simulink model "gm_sampleModel1695_sub"  (R2023a)
settings: Solver=VariableStepAuto  StartTime=0.0  StopTime=10.0  RelTol=1e-3
libraries: simulink x3
settings Model: Creator=user1  LastModifiedBy=user1
settings OptimizationCC: BlockReduction=off  ConditionallyExecuteInputs=off
settings DebuggingCC: InheritedTsInSrcMsg=none

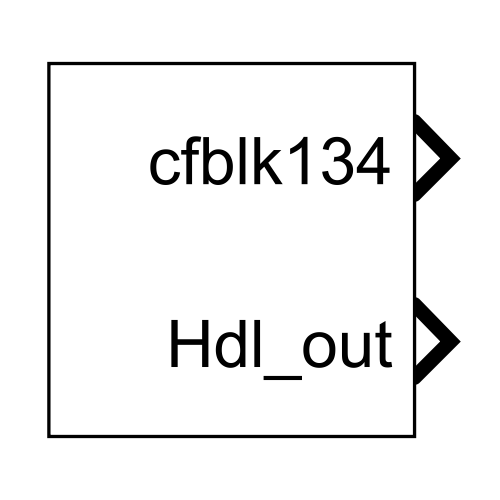
[thumbnail: Simulink's stored preview of the top-level diagram]
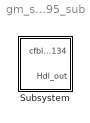
== system gm_sampleModel1695_sub ==
  Subsystem : Subsystem

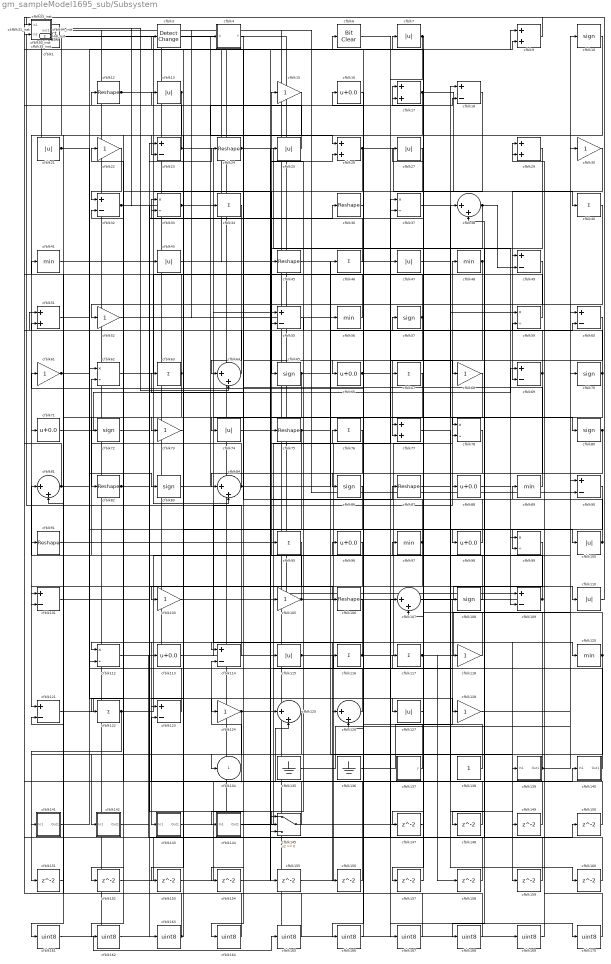
== system gm_sampleModel1695_sub/Subsystem ==
  cfblk1 : simulink/Logic and Bit Operations/Detect Increase  vinit=0.0  OutDataTypeStr=uint8
      settings: LibrarySourceBlock=|
      | hdlsllib/Logic and Bit
      | Operations/Detect
      | Increase
  cfblk{10,57,65,70,72,80,83,86,108} (9 alike) : Signum
  cfblk{7,13,21,25,27,43,47,74,100,110,115,127} (12 alike) : Abs  OutDataTypeStr=uint8  SaturateOnIntegerOverflow=off
  cfblk{18,23,32,49,55,60,69,90,101,109,114,121,123} (13 alike) : Sum  Inputs=+-  OutDataTypeStr=uint8
  cfblk102_inst : Subsystem
  cfblk{15,22,30,52,61,68,73,103,105,118,124,128} (12 alike) : Gain  OutDataTypeStr=uint8
  cfblk{12,24,36,45,75,82,87,91,106} (9 alike) : Reshape
  cfblk{38,64,81,84,107,125..126} (7 alike) : Sum  Inputs=|++  OutDataTypeStr=uint8
  cfblk{33,37,59,62,78,99,112} (7 alike) : Product  Inputs=*/  OutDataTypeStr=uint8  RndMeth=Zero  SaturateOnIntegerOverflow=on
  cfblk{16,66,71,88,96,98,113} (7 alike) : Bias  Bias=0.0  SaturateOnIntegerOverflow=off
  cfblk{34,40,46,63,67,76,95,116..117,122} (10 alike) : Sum  Inputs=+  OutDataTypeStr=uint8
  cfblk11_inst : Subsystem
  cfblk{41,48,56,89,97,120} (6 alike) : MinMax  OutDataTypeStr=uint8
  cfblk135 : Ground
  cfblk136 : Ground
  cfblk137 : Subsystem  mask(Counter Limited){uplimit=double(7), tsamp=double(-1)}
      mask prompts: uplimit "Simulink:masks:UpperLimit_MP"; tsamp "Simulink:masks:SampleTime_MP"
      mask help: Simulink:masks:CounterLimited_MD
      mask init:
      | nbits = double(8);
      | tsamp = double(-1);
      | uplimit = double(7);
  cfblk138 : Constant  OutDataTypeStr=uint8  SampleTime=-1
  cfblk139 : Subsystem
  cfblk140 : Subsystem
  cfblk141 : Subsystem
  cfblk142 : Subsystem
  cfblk143 : Subsystem
  cfblk144 : Subsystem
  cfblk145 : Switch  OutDataTypeStr=uint8  SaturateOnIntegerOverflow=off  InputSameDT=off
  cfblk{147..160} (14 alike) : Delay  SampleTime=1
  cfblk14_inst : Subsystem
  cfblk{161..170} (10 alike) : DataTypeConversion  OutDataTypeStr=uint8  SaturateOnIntegerOverflow=off  RndMeth=Floor
  cfblk{9,17,26,29,51,77} (6 alike) : Sum  OutDataTypeStr=uint8
  cfblk19_inst : Subsystem
  cfblk2 : Constant  Value=0  OutDataTypeStr=uint8  SampleTime=1
  cfblk28_inst : Subsystem
  cfblk3 : simulink/Logic and Bit Operations/Detect Change  vinit=0  OutDataTypeStr=uint8
      settings: LibrarySourceBlock=|
      | hdlsllib/Logic and Bit
      | Operations/Detect
      | Change
  cfblk31_inst : Subsystem
  cfblk35_inst : Subsystem
  cfblk4 : Subsystem  mask(Detect Fall Negative){vinit=double(0), InputProcessing=Elements as channels (sample based), OutDataTypeStr=uint8}
      mask prompts: vinit "Simulink:masks:InitialCondition_MP"; InputProcessing "Simulink:masks:InputProcessing_MP"; OutDataTypeStr "Simulink:masks:OutputDataType_MP"
      mask help: Simulink:masks:DetectFallNegative_MD
      mask init:
      | InputProcessing = 'Elements as channels (sample based)';
      | OutDataTypeStr = 'uint8';
      | vinit = double(0);
      mask TypeOptions InputProcessing: Simulink:masks:ColumnsAsChannelsFrameBased | Simulink:masks:ElementsAsChannelsSampleBased
      mask TypeOptions OutDataTypeStr: Simulink:masks:uint8 | Simulink:masks:boolean
      mask Display: fprintf('U < 0\n&  NOT\nU/z < 0')
  cfblk50_inst : Subsystem
  cfblk53_inst : Subsystem
  cfblk6 : simulink/Logic and Bit Operations/Bit Clear  iBit=0
      settings: LibrarySourceBlock=|
      | hdlsllib/Logic and Bit
      | Operations/Bit Clear
  cfblk94_inst : Subsystem
  cfblk134 : Outport  OutDataTypeStr=uint8  SampleTime=1  VectorParamsAs1DForOutWhenUnconnected=off
  Hdl_out : Outport  Port=2  OutDataTypeStr=uint8  SampleTime=1
  wires:
  cfblk1/1 -> cfblk84/2, cfblk121/1
  cfblk10/1 -> cfblk71/1
  cfblk100/1 -> cfblk48/1, cfblk89/1
  cfblk101/1 -> cfblk43/1
  cfblk102_inst/1(out1) -> cfblk47/1
  cfblk103/1 -> cfblk76/1
  cfblk105/1 -> cfblk81/1, cfblk15/1
  cfblk106/1 -> cfblk143/1(In1)
  cfblk107/1 -> cfblk110/1
  cfblk108/1 -> cfblk62/2
  cfblk109/1 -> cfblk91/1, Hdl_out/1
  cfblk11_inst/1(out1) -> cfblk109/1
  cfblk110/1 -> cfblk53_inst/1(in1)
  cfblk112/1 -> cfblk150/1
  cfblk113/1 -> cfblk88/1
  cfblk114/1 -> cfblk35_inst/2(in2)
  cfblk115/1 -> cfblk108/1, cfblk37/1
  cfblk116/1 -> cfblk78/2, cfblk112/1
  cfblk117/1 -> cfblk70/1, cfblk158/1
  cfblk118/1 -> cfblk33/1
  cfblk12/1 -> cfblk65/1, cfblk155/1
  cfblk120/1 -> cfblk31_inst/2(in2), cfblk142/1(In1)
  cfblk121/1 -> cfblk127/1
  cfblk122/1 -> cfblk151/1, cfblk97/1
  cfblk123/1 -> cfblk22/1
  cfblk124/1 -> cfblk134/1, cfblk117/1
  cfblk125/1 -> cfblk141/1(In1)
  cfblk126/1 -> cfblk3/1
  cfblk127/1 -> cfblk57/1
  cfblk128/1 -> cfblk30/1
  cfblk13/1 -> cfblk101/2, cfblk152/1
  cfblk135/1 -> cfblk10/1
  cfblk136/1 -> cfblk118/1
  cfblk137/1(y) -> cfblk96/1
  cfblk138/1 -> cfblk61/1
  cfblk139/1(Out1) -> cfblk90/1, cfblk75/1
  cfblk14_inst/1(out1) -> cfblk163/1
  cfblk140/1(Out1) -> cfblk62/1
  cfblk141/1(Out1) -> cfblk7/1
  cfblk142/1(Out1) -> cfblk140/1(In1)
  cfblk143/1(Out1) -> cfblk38/1
  cfblk144/1(Out1) -> cfblk46/1
  cfblk145/1 -> cfblk50_inst/2(in2)
  cfblk147/1 -> cfblk1/1
  cfblk148/1 -> cfblk51/2
  cfblk149/1 -> cfblk114/2
  cfblk15/1 -> cfblk23/2
  cfblk150/1 -> cfblk32/2
  cfblk151/1 -> cfblk121/2
  cfblk152/1 -> cfblk107/1
  cfblk153/1 -> cfblk125/2
  cfblk154/1 -> cfblk9/2
  cfblk155/1 -> cfblk60/1
  cfblk156/1 -> cfblk123/2
  cfblk157/1 -> cfblk17/1
  cfblk158/1 -> cfblk53_inst/2(in2)
  cfblk159/1 -> cfblk38/2
  cfblk16/1 -> cfblk66/1
  cfblk160/1 -> cfblk35_inst/1(in1)
  cfblk161/1 -> cfblk165/1
  cfblk162/1 -> cfblk95/1
  cfblk163/1 -> cfblk33/2, cfblk41/1
  cfblk164/1 -> cfblk14_inst/1(in1)
  cfblk165/1 -> cfblk14_inst/2(in2)
  cfblk166/1 -> cfblk6/1
  cfblk167/1 -> cfblk11_inst/2(in2)
  cfblk168/1 -> cfblk11_inst/1(in1)
  cfblk169/1 -> cfblk29/1
  cfblk17/1 -> cfblk69/2, cfblk103/1
  cfblk170/1 -> cfblk29/2
  cfblk18/1 -> cfblk45/1
  cfblk19_inst/1(out1) -> cfblk169/1
  cfblk2/1 -> cfblk64/2, cfblk4/1(U)
  cfblk21/1 -> cfblk9/1, cfblk124/1
  cfblk22/1 -> cfblk32/1
  cfblk23/1 -> cfblk12/1, cfblk156/1
  cfblk24/1 -> cfblk125/1, cfblk109/2
  cfblk25/1 -> cfblk28_inst/1(in1)
  cfblk26/1 -> cfblk73/1, cfblk40/1
  cfblk27/1 -> cfblk52/1
  cfblk28_inst/1(out1) -> cfblk56/1
  cfblk29/1 -> cfblk168/1
  cfblk3/1 -> cfblk26/1
  cfblk30/1 -> cfblk49/1
  cfblk31_inst/1(out1) -> cfblk90/2, cfblk28_inst/2(in2)
  cfblk32/1 -> cfblk126/1, cfblk106/1
  cfblk33/1 -> cfblk77/2, cfblk55/1, cfblk159/1, cfblk105/1
  cfblk34/1 -> cfblk64/1
  cfblk35_inst/1(out1) -> cfblk113/1
  cfblk36/1 -> cfblk16/1
  cfblk37/1 -> cfblk59/1
  cfblk38/1 -> cfblk55/2, cfblk49/2
  cfblk4/1(Y) -> cfblk164/1
  cfblk40/1 -> cfblk122/1
  cfblk41/1 -> cfblk98/1
  cfblk43/1 -> cfblk18/2
  cfblk45/1 -> cfblk78/1
  cfblk46/1 -> cfblk23/1
  cfblk47/1 -> cfblk80/1
  cfblk48/1 -> cfblk77/1, cfblk126/2
  cfblk49/1 -> cfblk114/1
  cfblk50_inst/1(out1) -> cfblk115/1
  cfblk51/1 -> cfblk83/1
  cfblk52/1 -> cfblk26/2
  cfblk53_inst/1(out1) -> cfblk34/1
  cfblk55/1 -> cfblk145/2
  cfblk56/1 -> cfblk102_inst/1(in1)
  cfblk57/1 -> cfblk19_inst/2(in2), cfblk67/1
  cfblk59/1 -> cfblk27/1
  cfblk6/1 -> cfblk167/1
  cfblk60/1 -> cfblk144/1(In1)
  cfblk61/1 -> cfblk100/1, cfblk128/1
  cfblk62/1 -> cfblk18/1
  cfblk63/1 -> cfblk94_inst/2(in2), cfblk82/1
  cfblk64/1 -> cfblk51/1
  cfblk65/1 -> cfblk101/1, cfblk139/1(In1)
  cfblk66/1 -> cfblk170/1, cfblk68/1
  cfblk67/1 -> cfblk123/1
  cfblk68/1 -> cfblk116/1
  cfblk69/1 -> cfblk94_inst/1(in1), cfblk147/1
  cfblk7/1 -> cfblk107/2, cfblk37/2
  cfblk70/1 -> cfblk81/2, cfblk74/1, cfblk25/1
  cfblk71/1 -> cfblk69/1
  cfblk72/1 -> cfblk36/1
  cfblk73/1 -> cfblk13/1
  cfblk74/1 -> cfblk120/1
  cfblk75/1 -> cfblk59/2, cfblk153/1
  cfblk76/1 -> cfblk86/1
  cfblk77/1 -> cfblk160/1
  cfblk78/1 -> cfblk166/1
  cfblk80/1 -> cfblk84/1, cfblk148/1
  cfblk81/1 -> cfblk50_inst/1(in1), cfblk99/2
  cfblk82/1 -> cfblk24/1, cfblk145/3
  cfblk83/1 -> cfblk17/2
  cfblk84/1 -> cfblk72/1, cfblk60/2
  cfblk86/1 -> cfblk145/1
  cfblk87/1 -> cfblk149/1
  cfblk88/1 -> cfblk99/1
  cfblk89/1 -> cfblk102_inst/2(in2)
  cfblk9/1 -> cfblk31_inst/1(in1)
  cfblk90/1 -> cfblk154/1
  cfblk91/1 -> cfblk87/1
  cfblk94_inst/1(out1) -> cfblk21/1
  cfblk95/1 -> cfblk161/1
  cfblk96/1 -> cfblk162/1
  cfblk97/1 -> cfblk19_inst/1(in1), cfblk112/2
  cfblk98/1 -> cfblk63/1
  cfblk99/1 -> cfblk157/1

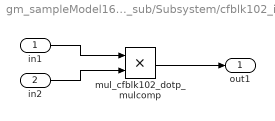
== system gm_sampleModel1695_sub/Subsystem/cfblk102_inst ==
  in1 : Inport  OutDataTypeStr=uint8  SampleTime=1
  in2 : Inport  Port=2  OutDataTypeStr=uint8  SampleTime=1
  mul_cfblk102_dotp_mulcomp : Product  Inputs=**  OutDataTypeStr=uint8  SampleTime=1
  out1 : Outport  OutDataTypeStr=uint8  SampleTime=1
  wires:
  in1/1 -> mul_cfblk102_dotp_mulcomp/1
  in2/1 -> mul_cfblk102_dotp_mulcomp/2
  mul_cfblk102_dotp_mulcomp/1 -> out1/1

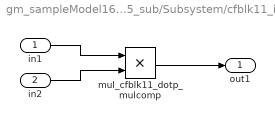
== system gm_sampleModel1695_sub/Subsystem/cfblk11_inst ==
  in1 : Inport  OutDataTypeStr=uint8  SampleTime=1
  in2 : Inport  Port=2  OutDataTypeStr=uint8  SampleTime=1
  mul_cfblk11_dotp_mulcomp : Product  Inputs=**  OutDataTypeStr=uint8  SampleTime=1
  out1 : Outport  OutDataTypeStr=uint8  SampleTime=1
  wires:
  in1/1 -> mul_cfblk11_dotp_mulcomp/1
  in2/1 -> mul_cfblk11_dotp_mulcomp/2
  mul_cfblk11_dotp_mulcomp/1 -> out1/1

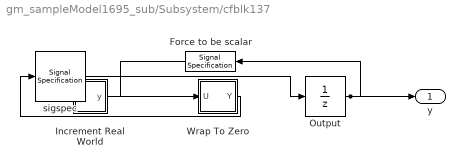
== system gm_sampleModel1695_sub/Subsystem/cfblk137 ==
  Force to be scalar : SignalSpecification  DisableCoverage=on  Dimensions=1
  Increment Real World : Subsystem  mask(Real World Value Increment){}
      mask help: Simulink:masks:RealWorldValueIncrement_MD
      mask Display: disp('V++')
  Output : UnitDelay  InitialCondition=0.0  SampleTime=tsamp  HasFrameUpgradeWarning=on
  Wrap To Zero : Subsystem  mask(Wrap To Zero){Threshold=double(7)}
      mask prompts: Threshold "Simulink:masks:Threshold_MP"
      mask help: Simulink:masks:WrapToZero_MD
  sigspec : SignalSpecification  OutDataTypeStr=uint8  Dimensions=1
  y : Outport  SampleTime=1
  wires:
  Force to be scalar/1 -> Increment Real World/1(u)
  Increment Real World/1(y) -> Wrap To Zero/1(U)
  Output/1 -> Force to be scalar/1, y/1
  Wrap To Zero/1(Y) -> sigspec/1
  sigspec/1 -> Output/1

== system gm_sampleModel1695_sub/Subsystem/cfblk139 ==
  In1 : Inport  OutDataTypeStr=uint8  PortDimensions=1  SampleTime=1
  Out1 : Outport  SampleTime=1
  wires:
  In1/1 -> Out1/1

== system gm_sampleModel1695_sub/Subsystem/cfblk140 ==
  In1 : Inport  OutDataTypeStr=uint8  PortDimensions=1  SampleTime=1
  Out1 : Outport  SampleTime=1
  wires:
  In1/1 -> Out1/1

== system gm_sampleModel1695_sub/Subsystem/cfblk141 ==
  In1 : Inport  OutDataTypeStr=uint8  PortDimensions=1  SampleTime=1
  Out1 : Outport  SampleTime=1
  wires:
  In1/1 -> Out1/1

== system gm_sampleModel1695_sub/Subsystem/cfblk142 ==
  In1 : Inport  OutDataTypeStr=uint8  PortDimensions=1  SampleTime=1
  Out1 : Outport  SampleTime=1
  wires:
  In1/1 -> Out1/1

== system gm_sampleModel1695_sub/Subsystem/cfblk143 ==
  In1 : Inport  OutDataTypeStr=uint8  PortDimensions=1  SampleTime=1
  Out1 : Outport  SampleTime=1
  wires:
  In1/1 -> Out1/1

== system gm_sampleModel1695_sub/Subsystem/cfblk144 ==
  In1 : Inport  OutDataTypeStr=uint8  PortDimensions=1  SampleTime=1
  Out1 : Outport  SampleTime=1
  wires:
  In1/1 -> Out1/1

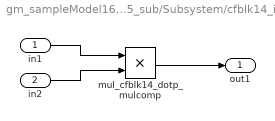
== system gm_sampleModel1695_sub/Subsystem/cfblk14_inst ==
  in1 : Inport  OutDataTypeStr=uint8  SampleTime=1
  in2 : Inport  Port=2  OutDataTypeStr=uint8  SampleTime=1
  mul_cfblk14_dotp_mulcomp : Product  Inputs=**  OutDataTypeStr=uint8  SampleTime=1
  out1 : Outport  OutDataTypeStr=uint8  SampleTime=1
  wires:
  in1/1 -> mul_cfblk14_dotp_mulcomp/1
  in2/1 -> mul_cfblk14_dotp_mulcomp/2
  mul_cfblk14_dotp_mulcomp/1 -> out1/1

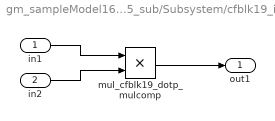
== system gm_sampleModel1695_sub/Subsystem/cfblk19_inst ==
  in1 : Inport  OutDataTypeStr=uint8  SampleTime=1
  in2 : Inport  Port=2  OutDataTypeStr=uint8  SampleTime=1
  mul_cfblk19_dotp_mulcomp : Product  Inputs=**  OutDataTypeStr=uint8  SampleTime=1
  out1 : Outport  OutDataTypeStr=uint8  SampleTime=1
  wires:
  in1/1 -> mul_cfblk19_dotp_mulcomp/1
  in2/1 -> mul_cfblk19_dotp_mulcomp/2
  mul_cfblk19_dotp_mulcomp/1 -> out1/1

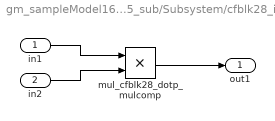
== system gm_sampleModel1695_sub/Subsystem/cfblk28_inst ==
  in1 : Inport  OutDataTypeStr=uint8  SampleTime=1
  in2 : Inport  Port=2  OutDataTypeStr=uint8  SampleTime=1
  mul_cfblk28_dotp_mulcomp : Product  Inputs=**  OutDataTypeStr=uint8  SampleTime=1
  out1 : Outport  OutDataTypeStr=uint8  SampleTime=1
  wires:
  in1/1 -> mul_cfblk28_dotp_mulcomp/1
  in2/1 -> mul_cfblk28_dotp_mulcomp/2
  mul_cfblk28_dotp_mulcomp/1 -> out1/1

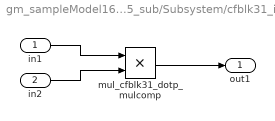
== system gm_sampleModel1695_sub/Subsystem/cfblk31_inst ==
  in1 : Inport  OutDataTypeStr=uint8  SampleTime=1
  in2 : Inport  Port=2  OutDataTypeStr=uint8  SampleTime=1
  mul_cfblk31_dotp_mulcomp : Product  Inputs=**  OutDataTypeStr=uint8  SampleTime=1
  out1 : Outport  OutDataTypeStr=uint8  SampleTime=1
  wires:
  in1/1 -> mul_cfblk31_dotp_mulcomp/1
  in2/1 -> mul_cfblk31_dotp_mulcomp/2
  mul_cfblk31_dotp_mulcomp/1 -> out1/1

== system gm_sampleModel1695_sub/Subsystem/cfblk35_inst ==
  in1 : Inport  OutDataTypeStr=uint8  SampleTime=1
  in2 : Inport  Port=2  OutDataTypeStr=uint8  SampleTime=1
  mul_cfblk35_dotp_mulcomp : Product  Inputs=**  OutDataTypeStr=uint8  SampleTime=1
  out1 : Outport  OutDataTypeStr=uint8  SampleTime=1
  wires:
  in1/1 -> mul_cfblk35_dotp_mulcomp/1
  in2/1 -> mul_cfblk35_dotp_mulcomp/2
  mul_cfblk35_dotp_mulcomp/1 -> out1/1

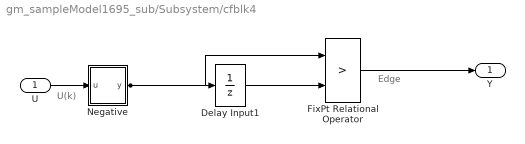
== system gm_sampleModel1695_sub/Subsystem/cfblk4 ==
  note: U(k)
  note: Edge
  U : Inport  OutDataTypeStr=uint8  SampleTime=1
  Delay Input1 : UnitDelay  Description=Store in Global RAM  DisableCoverage=on  InitialCondition=vinit  SampleTime=-1  HasFrameUpgradeWarning=on
  FixPt Relational Operator : RelationalOperator  Operator=>  OutDataTypeStr=fixdt(0, 8)  ZeroCross=off  InputSameDT=off
  Negative : Subsystem  mask(Compare To Zero){relop=<, OutDataTypeStr=boolean, ZeroCross=off}
      mask prompts: relop "Simulink:masks:Operator_MP"; OutDataTypeStr "Simulink:masks:OutputDataType_MP"; ZeroCross "Simulink:masks:EnableZerocrossingDetection_MP"
      mask help: Simulink:masks:CompareToZero_MD
      mask init:
      | OutDataTypeStr = 'boolean';
      | ZeroCross = 'off';
      | blkName = 'sampleModel1695_sub/Subsystem/cfblk4/Negative';
      | relop = '<';
      | setValue = 'boolean';
      mask TypeOptions relop: == | ~= | < | <= | >= | >
      mask TypeOptions OutDataTypeStr: Simulink:masks:uint8 | Simulink:masks:boolean
      mask Callback ZeroCross: sl('zeroCrossEnable', gcbh);
      mask Display: disp([relop,' 0'])
  Y : Outport  SampleTime=1
  wires:
  U/1 -> Negative/1(u)
  Delay Input1/1 -> FixPt Relational Operator/2
  FixPt Relational Operator/1 -> Y/1
  Negative/1(y) -> FixPt Relational Operator/1, Delay Input1/1

== system gm_sampleModel1695_sub/Subsystem/cfblk50_inst ==
  in1 : Inport  OutDataTypeStr=uint8  SampleTime=1
  in2 : Inport  Port=2  OutDataTypeStr=uint8  SampleTime=1
  mul_cfblk50_dotp_mulcomp : Product  Inputs=**  OutDataTypeStr=uint8  SampleTime=1
  out1 : Outport  OutDataTypeStr=uint8  SampleTime=1
  wires:
  in1/1 -> mul_cfblk50_dotp_mulcomp/1
  in2/1 -> mul_cfblk50_dotp_mulcomp/2
  mul_cfblk50_dotp_mulcomp/1 -> out1/1

== system gm_sampleModel1695_sub/Subsystem/cfblk53_inst ==
  in1 : Inport  OutDataTypeStr=uint8  SampleTime=1
  in2 : Inport  Port=2  OutDataTypeStr=uint8  SampleTime=1
  mul_cfblk53_dotp_mulcomp : Product  Inputs=**  OutDataTypeStr=uint8  SampleTime=1
  out1 : Outport  OutDataTypeStr=uint8  SampleTime=1
  wires:
  in1/1 -> mul_cfblk53_dotp_mulcomp/1
  in2/1 -> mul_cfblk53_dotp_mulcomp/2
  mul_cfblk53_dotp_mulcomp/1 -> out1/1

== system gm_sampleModel1695_sub/Subsystem/cfblk94_inst ==
  in1 : Inport  OutDataTypeStr=uint8  SampleTime=1
  in2 : Inport  Port=2  OutDataTypeStr=uint8  SampleTime=1
  mul_cfblk94_dotp_mulcomp : Product  Inputs=**  OutDataTypeStr=uint8  SampleTime=1
  out1 : Outport  OutDataTypeStr=uint8  SampleTime=1
  wires:
  in1/1 -> mul_cfblk94_dotp_mulcomp/1
  in2/1 -> mul_cfblk94_dotp_mulcomp/2
  mul_cfblk94_dotp_mulcomp/1 -> out1/1

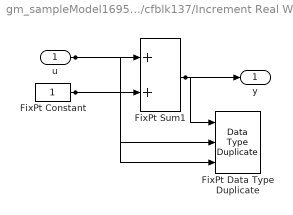
== system gm_sampleModel1695_sub/Subsystem/cfblk137/Increment Real World ==
  u : Inport  OutDataTypeStr=uint8  SampleTime=1
  FixPt Constant : Constant  DisableCoverage=on  OutDataTypeStr=Inherit: Inherit via back propagation  SampleTime=-1
  FixPt Data Type Duplicate : DataTypeDuplicate  DisableCoverage=on  NumInputPorts=3
  FixPt Sum1 : Sum  InputSameDT=on  OutDataTypeStr=Inherit: Inherit via back propagation  LockScale=on
  y : Outport  SampleTime=1
  wires:
  u/1 -> FixPt Sum1/1, FixPt Data Type Duplicate/2
  FixPt Constant/1 -> FixPt Sum1/2, FixPt Data Type Duplicate/3
  FixPt Sum1/1 -> FixPt Data Type Duplicate/1, y/1

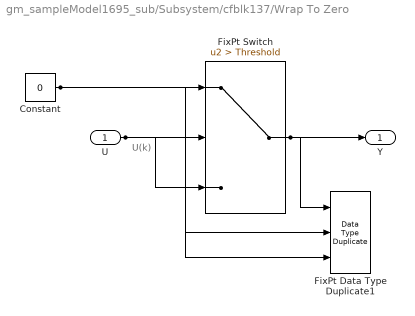
== system gm_sampleModel1695_sub/Subsystem/cfblk137/Wrap To Zero ==
  note: U(k)
  U : Inport  OutDataTypeStr=uint8  SampleTime=1
  Constant : Constant  DisableCoverage=on  Value=0  OutDataTypeStr=Inherit: Inherit via back propagation  SampleTime=-1
  FixPt Data Type Duplicate1 : DataTypeDuplicate  DisableCoverage=on  NumInputPorts=3
  FixPt Switch : Switch  Criteria=u2 > Threshold  Threshold=Threshold  OutDataTypeStr=Inherit: Inherit via back propagation  ZeroCross=off  SaturateOnIntegerOverflow=off  InputSameDT=off
  Y : Outport  SampleTime=1
  wires:
  U/1 -> FixPt Switch/3, FixPt Switch/2, FixPt Data Type Duplicate1/2
  Constant/1 -> FixPt Switch/1, FixPt Data Type Duplicate1/3
  FixPt Switch/1 -> FixPt Data Type Duplicate1/1, Y/1

== system gm_sampleModel1695_sub/Subsystem/cfblk4/Negative ==
  u : Inport  OutDataTypeStr=uint8  SampleTime=1
  Compare : RelationalOperator  Operator=<  OutDataTypeStr=boolean  ZeroCross=off
  Constant : Constant  DisableCoverage=on  Value=0  OutDataTypeStr=Inherit: Inherit via back propagation  SampleTime=-1  PreserveConstantTs=on
  y : Outport  SampleTime=1
  wires:
  u/1 -> Compare/1
  Compare/1 -> y/1
  Constant/1 -> Compare/2
